simulink model "Moteur_Complet"  (Simulink 10.1)
settings: Solver=ode45  StartTime=0.0  StopTime=T_Sim  MaxStep=T_s  RelTol=1e-3  EnableMultiTasking=on
values from neighbouring files (symbols this model uses):
  a0 = Te-2*T3    (= -0.00375)    [BE_Chaines.m]
  a1 = Te+2*T3    (= 0.00425)    [BE_Chaines.m]
  b0 = -2*T4    (= -0.00579332424904)    [BE_Chaines.m]
  b1 = 2*T4    (= 0.00579332424904)    [BE_Chaines.m]
  Den_C = [T4 0]    [BE_Chaines.m]
  Den_Elec = [T0 1]    [BE_Chaines.m]    (also in Param_Moteur.m = [L/R 1])
  Den_F = [T1*T2 T1+T2 1]    [BE_Chaines.m]
  Den_Meca = [Jeq/fv 1]    [BE_Chaines.m]    (also in Param_Moteur.m)
  I0 = 1    [BE_Chaines.m]
  K_C1 = RRoue*(R1/R2)*M*g*(pi/180)/n    (= 0.145534279678)    [BE_Chaines.m]    (also in Param_Moteur.m)
  KI = 76e-3    (= 0.076)    [BE_Chaines.m]    (also in Param_Moteur.m)
  Kretour = G1    (= 0.151668874172)    [BE_Chaines.m]
  Num_C = [T3 1]    [BE_Chaines.m]
  Num_Elec = G0    (= 48)    [BE_Chaines.m]    (also in Param_Moteur.m = 0.833333333333)
  Num_F = Kmef*Si    (= 0.151668874172)    [BE_Chaines.m]
  Num_Meca = 1/fv    (= 4000)    [BE_Chaines.m]    (also in Param_Moteur.m)
  Te = 1/fe    (= 0.00025)    [BE_Chaines.m]
settings Model: Creator=trocache  LastModifiedBy=moumen
settings DataIOCC: LimitDataPoints=on  SignalLoggingSaveFormat=ModelDataLogs
settings OptimizationCC: ExpressionDepthLimit=2147483647
settings DebuggingCC: FcnCallInpInsideContextMsg=warning  StateNameClashWarn=warning
settings GRTTargetCC: CombineOutputUpdateFcns=on  GRTInterface=off

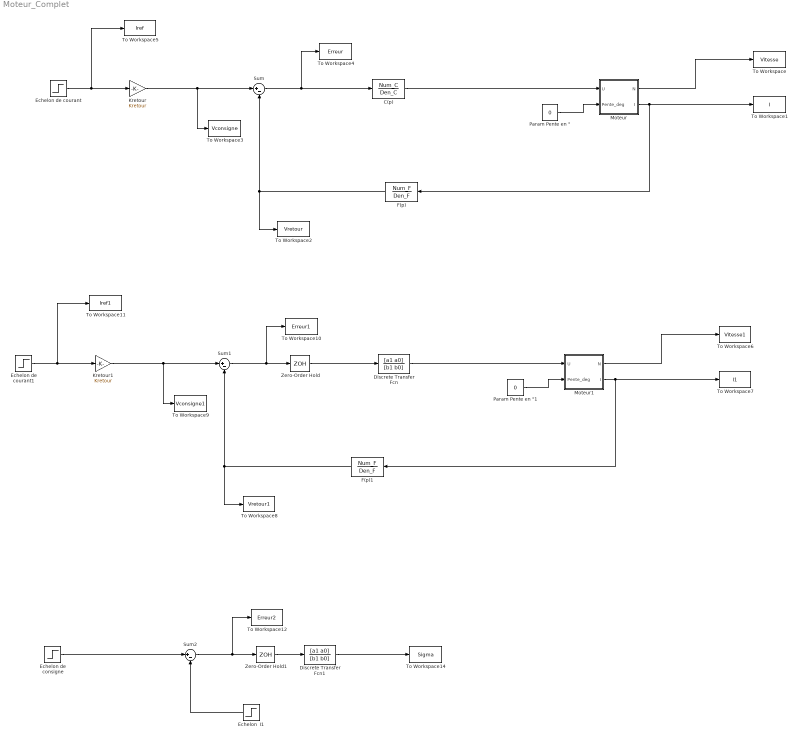
== system Moteur_Complet ==
  C(p) : TransferFcn  Numerator=Num_C  Denominator=Den_C
  Discrete Transfer Fcn : DiscreteTransferFcn  Numerator=[a1 a0]  Denominator=[b1 b0]
  Discrete Transfer Fcn1 : DiscreteTransferFcn  Numerator=[a1 a0]  Denominator=[b1 b0]
  Echelon  I1 : Step  Time=0  After=1.65  SampleTime=0
  Echelon de consigne : Step  Time=0  After=1.75  SampleTime=0
  Echelon de courant : Step  Time=0  After=I0  SampleTime=0
  Echelon de courant1 : Step  Time=0  After=I0  SampleTime=0
  F(p) : TransferFcn  Numerator=Num_F  Denominator=Den_F
  F(p)1 : TransferFcn  Numerator=Num_F  Denominator=Den_F
  Kretour : Gain  Gain=Kretour
  Kretour1 : Gain  Gain=Kretour
  Moteur : Subsystem
  Moteur1 : Subsystem
  Param Pente en ° : Constant  Value=0
  Param Pente en °1 : Constant  Value=0
  Sum : Sum  Inputs=|+-
  Sum1 : Sum  Inputs=|+-
  Sum2 : Sum  Inputs=|+-
  To Workspace : ToWorkspace  VariableName=Vitesse  SaveFormat=Structure With Time  SampleTime=-1
  To Workspace1 : ToWorkspace  VariableName=I  SaveFormat=Structure With Time  SampleTime=-1
  To Workspace10 : ToWorkspace  VariableName=Erreur1  SaveFormat=Structure With Time  SampleTime=-1
  To Workspace11 : ToWorkspace  VariableName=Iref1  SaveFormat=Structure With Time  SampleTime=-1
  To Workspace12 : ToWorkspace  VariableName=Erreur2  SaveFormat=Structure With Time  SampleTime=-1
  To Workspace14 : ToWorkspace  VariableName=Sigma  SaveFormat=Structure With Time  SampleTime=-1
  To Workspace2 : ToWorkspace  VariableName=Vretour  SaveFormat=Structure With Time  SampleTime=-1
  To Workspace3 : ToWorkspace  VariableName=Vconsigne  SaveFormat=Structure With Time  SampleTime=-1
  To Workspace4 : ToWorkspace  VariableName=Erreur  SaveFormat=Structure With Time  SampleTime=-1
  To Workspace5 : ToWorkspace  VariableName=Iref  SaveFormat=Structure With Time  SampleTime=-1
  To Workspace6 : ToWorkspace  VariableName=Vitesse1  SaveFormat=Structure With Time  SampleTime=-1
  To Workspace7 : ToWorkspace  VariableName=I1  SaveFormat=Structure With Time  SampleTime=-1
  To Workspace8 : ToWorkspace  VariableName=Vretour1  SaveFormat=Structure With Time  SampleTime=-1
  To Workspace9 : ToWorkspace  VariableName=Vconsigne1  SaveFormat=Structure With Time  SampleTime=-1
  Zero-Order Hold : ZeroOrderHold  SampleTime=Te
  Zero-Order Hold1 : ZeroOrderHold  SampleTime=Te
  wires:
  Param Pente en °/1 -> Moteur/2(Pente_deg)
  Moteur/1(N) -> To Workspace/1
  Moteur/2(I) -> F(p)/1, To Workspace1/1
  Echelon de courant/1 -> To Workspace5/1, Kretour/1
  Sum/1 -> To Workspace4/1, C(p)/1
  C(p)/1 -> Moteur/1(U)
  F(p)/1 -> To Workspace2/1, Sum/2
  Kretour/1 -> To Workspace3/1, Sum/1
  F(p)1/1 -> To Workspace8/1, Sum1/2
  Kretour1/1 -> To Workspace9/1, Sum1/1
  Echelon de courant1/1 -> To Workspace11/1, Kretour1/1
  Moteur1/2(I) -> F(p)1/1, To Workspace7/1
  Moteur1/1(N) -> To Workspace6/1
  Discrete Transfer Fcn/1 -> Moteur1/1(U)
  Sum1/1 -> Zero-Order Hold/1, To Workspace10/1
  Param Pente en °1/1 -> Moteur1/2(Pente_deg)
  Zero-Order Hold/1 -> Discrete Transfer Fcn/1
  Echelon  I1/1 -> Sum2/2
  Echelon de consigne/1 -> Sum2/1
  Zero-Order Hold1/1 -> Discrete Transfer Fcn1/1
  Sum2/1 -> Zero-Order Hold1/1, To Workspace12/1
  Discrete Transfer Fcn1/1 -> To Workspace14/1

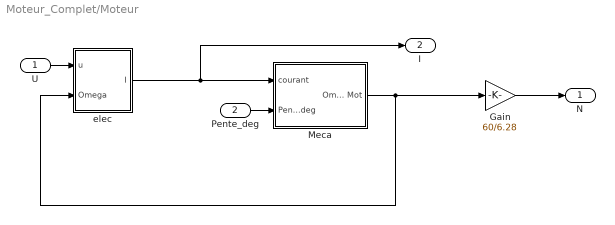
== system Moteur_Complet/Moteur ==
  U : Inport
  Pente_deg : Inport  Port=2
  Gain : Gain  Gain=60/6.28
  Meca : Subsystem
  elec : Subsystem
  N : Outport
  I : Outport  Port=2
  wires:
  Meca/1(Omega Mot) -> elec/2(Omega), Gain/1
  elec/1(I) -> Meca/1(courant), I/1
  U/1 -> elec/1(u)
  Pente_deg/1 -> Meca/2(Pente_deg)
  Gain/1 -> N/1

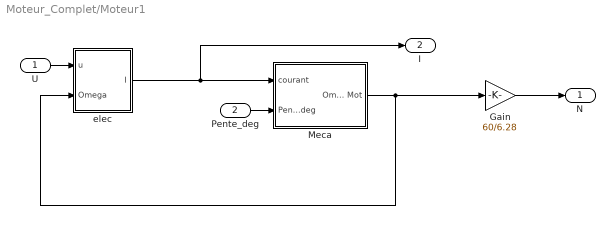
== system Moteur_Complet/Moteur1 ==
  U : Inport
  Pente_deg : Inport  Port=2
  Gain : Gain  Gain=60/6.28
  Meca : Subsystem
  elec : Subsystem
  N : Outport
  I : Outport  Port=2
  wires:
  Meca/1(Omega Mot) -> elec/2(Omega), Gain/1
  elec/1(I) -> Meca/1(courant), I/1
  U/1 -> elec/1(u)
  Pente_deg/1 -> Meca/2(Pente_deg)
  Gain/1 -> N/1

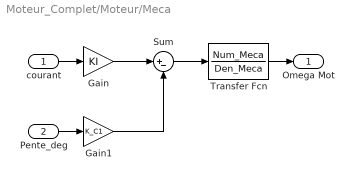
== system Moteur_Complet/Moteur/Meca ==
  courant : Inport
  Pente_deg : Inport  Port=2
  Gain : Gain  Gain=KI
  Gain1 : Gain  Gain=K_C1
  Sum : Sum  Inputs=|+-
  Transfer Fcn : TransferFcn  Numerator=Num_Meca  Denominator=Den_Meca
  Omega Mot : Outport
  wires:
  Sum/1 -> Transfer Fcn/1
  Gain/1 -> Sum/1
  courant/1 -> Gain/1
  Transfer Fcn/1 -> Omega Mot/1
  Pente_deg/1 -> Gain1/1
  Gain1/1 -> Sum/2

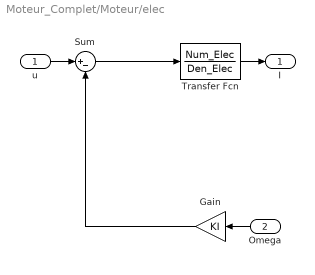
== system Moteur_Complet/Moteur/elec ==
  u : Inport
  Omega : Inport  Port=2
  Gain : Gain  Gain=KI
  Sum : Sum  Inputs=|+-
  Transfer Fcn : TransferFcn  Numerator=Num_Elec  Denominator=Den_Elec
  I : Outport
  wires:
  Sum/1 -> Transfer Fcn/1
  Gain/1 -> Sum/2
  u/1 -> Sum/1
  Transfer Fcn/1 -> I/1
  Omega/1 -> Gain/1

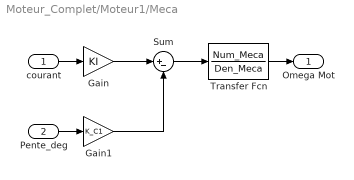
== system Moteur_Complet/Moteur1/Meca ==
  courant : Inport
  Pente_deg : Inport  Port=2
  Gain : Gain  Gain=KI
  Gain1 : Gain  Gain=K_C1
  Sum : Sum  Inputs=|+-
  Transfer Fcn : TransferFcn  Numerator=Num_Meca  Denominator=Den_Meca
  Omega Mot : Outport
  wires:
  Sum/1 -> Transfer Fcn/1
  Gain/1 -> Sum/1
  courant/1 -> Gain/1
  Transfer Fcn/1 -> Omega Mot/1
  Pente_deg/1 -> Gain1/1
  Gain1/1 -> Sum/2

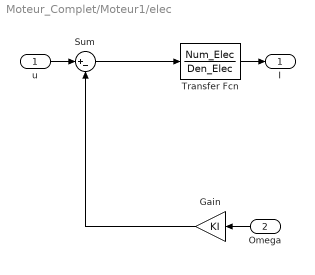
== system Moteur_Complet/Moteur1/elec ==
  u : Inport
  Omega : Inport  Port=2
  Gain : Gain  Gain=KI
  Sum : Sum  Inputs=|+-
  Transfer Fcn : TransferFcn  Numerator=Num_Elec  Denominator=Den_Elec
  I : Outport
  wires:
  Sum/1 -> Transfer Fcn/1
  Gain/1 -> Sum/2
  u/1 -> Sum/1
  Transfer Fcn/1 -> I/1
  Omega/1 -> Gain/1
